simulink model "untitled"  (R2018a)
settings: Solver=VariableStepAuto  StartTime=0.0  StopTime=12  RelTol=1e-3
values from neighbouring files (symbols this model uses):
  g = 9.81    [Untitled.m]
  K_R = 0.5    [Untitled.m]
  T_1 = 0.1    [Untitled.m]
  T_D = 1    [Untitled.m]
  x0 = 0.3    [Untitled.m]
settings Model: Creator=Hoursana  LastModifiedBy=Hoursana

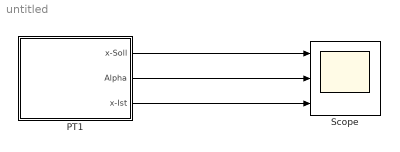
== system untitled ==
  PT1 : Subsystem
  Scope : Scope  NumInputPorts=3
  wires:
  PT1/1(x-Soll) -> Scope/1
  PT1/2(Alpha) -> Scope/2
  PT1/3(x-Ist) -> Scope/3

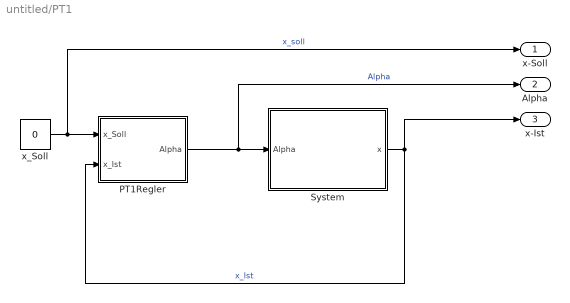
== system untitled/PT1 ==
  " PT1Regler" : Subsystem
  System : Subsystem  TreatAsAtomicUnit=on
  x_Soll : Constant  Value=0
  x-Soll : Outport
  Alpha : Outport  Port=2
  x-Ist : Outport  Port=3
  wires:
  " PT1Regler"/1(Alpha) -> System/1(Alpha), Alpha/1  "Alpha"
  System/1(x) -> " PT1Regler"/2(x_Ist), x-Ist/1  "x_Ist"
  x_Soll/1 -> x-Soll/1, " PT1Regler"/1(x_Soll)  "x_soll"

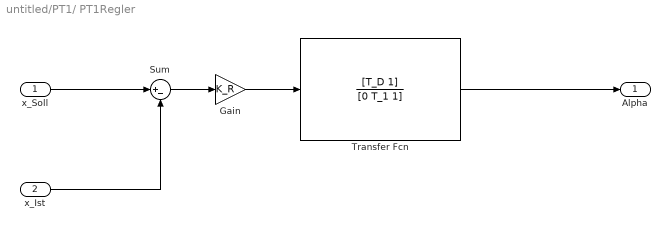
== system untitled/PT1/ PT1Regler ==
  x_Soll : Inport
  x_Ist : Inport  Port=2
  Gain : Gain  Gain=K_R
  Sum : Sum  Inputs=|+-
  Transfer Fcn : TransferFcn  Numerator=[T_D 1]  Denominator=[0 T_1 1]
  Alpha : Outport
  wires:
  x_Soll/1 -> Sum/1
  x_Ist/1 -> Sum/2
  Sum/1 -> Gain/1
  Transfer Fcn/1 -> Alpha/1
  Gain/1 -> Transfer Fcn/1

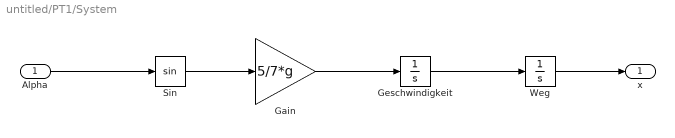
== system untitled/PT1/System ==
  Alpha : Inport
  Gain : Gain  Gain=5/7*g
  Geschwindigkeit : Integrator
  Sin : Trigonometry
  Weg : Integrator  InitialCondition=x0
  x : Outport
  wires:
  Alpha/1 -> Sin/1
  Weg/1 -> x/1
  Gain/1 -> Geschwindigkeit/1
  Geschwindigkeit/1 -> Weg/1
  Sin/1 -> Gain/1
